simulink model "Generator1"  (Simulink 7.6)
settings: Solver=FixedStepDiscrete  StartTime=0.0  StopTime=1  FixedStep=1  RelTol=1e-3
libraries: simulink x2
settings Model: Creator=jordan  LastModifiedBy=jordan
settings OptimizationCC: BlockReduction=off  ConditionallyExecuteInputs=off  InlineParams=on

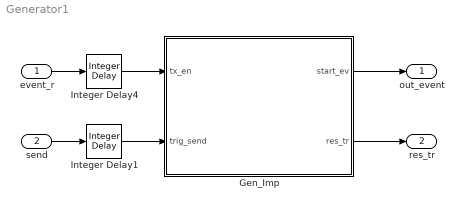
== system Generator1 ==
  event_r : Inport  OutDataTypeStr=boolean
  send : Inport  Port=2  OutDataTypeStr=boolean
  Gen_Imp : Stateflow chart  TreatAsAtomicUnit=on
  Integer Delay1 : simulink/Discrete/Integer Delay  NumDelays=1  vinit=0.0  samptime=-1
  Integer Delay4 : simulink/Discrete/Integer Delay  NumDelays=1  vinit=0.0  samptime=-1
  out_event : Outport  OutDataTypeStr=boolean
  res_tr : Outport  Port=2  OutDataTypeStr=boolean
  wires:
  event_r/1 -> Integer Delay4/1
  Gen_Imp/1(start_ev) -> out_event/1
  Integer Delay4/1 -> Gen_Imp/1(tx_en)
  Gen_Imp/2(res_tr) -> res_tr/1
  send/1 -> Integer Delay1/1
  Integer Delay1/1 -> Gen_Imp/2(trig_send)

== stateflow chart Gen_Imp ==
  settings: executeAtInitialization=1
  state Wait1
  state Start
  state Wait
  state Reset
  state Wait3
  (default) -> Wait
  Start -> Wait1 : [tx_en==1]{
      | acc=0;
      | start_ev=0;}
  (junction 9) -> (junction 11) [order 1] : [tx_en==0]
  Wait -> (junction 8)
  (junction 8) -> Wait [order 1] : [acc<1000]{acc++;}
  Wait3 -> Start : [trig_send==1]{start_ev=1;}
  (junction 10) -> Reset [order 2] : {res_tr=1;}
  (junction 9) -> Wait1 [order 2]
  Reset -> (junction 11) : {res_tr=0;}
  (junction 10) -> (junction 9) [order 1] : [acc<100000000]{
      | acc++;}
  Wait1 -> (junction 10)
  (junction 11) -> Wait : {acc=0;}
  (junction 8) -> Wait3 [order 2]
  data: tx_en input boolean; start_ev output boolean; acc local uint32 =0; res_tr output boolean =0; trig_send input boolean
